simulink model "B12U_HVDC"  (R2024a)
settings: Solver=VariableStepAuto  StartTime=0.0  StopTime=0.02  MaxStep=1e-5  RelTol=1e-3
undefined symbols (not defined in the file or in its folder): D1, Delta
libraries: spsDiodeLib x12, spsVoltageMeasurementLib x7, spsACVoltageSourceLib x3, spsCurrentMeasurementLib x1, spsGroundLib x1, spsSeriesRLCBranchLib x1, spsThreePhaseTransformerThreeWindingsLib x1, sps_lib x1
settings Model: Creator=E370_  LastModifiedBy=E370_

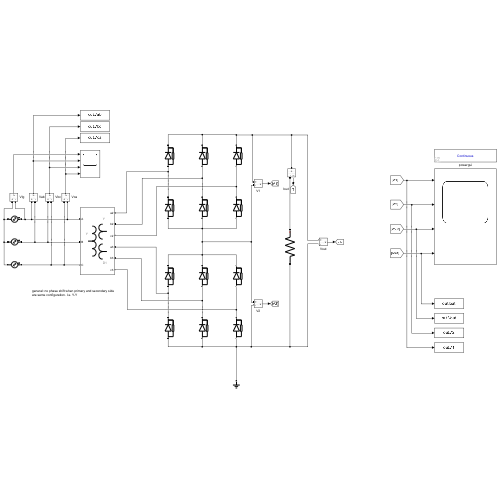
[thumbnail: Simulink's stored preview of the top-level diagram]
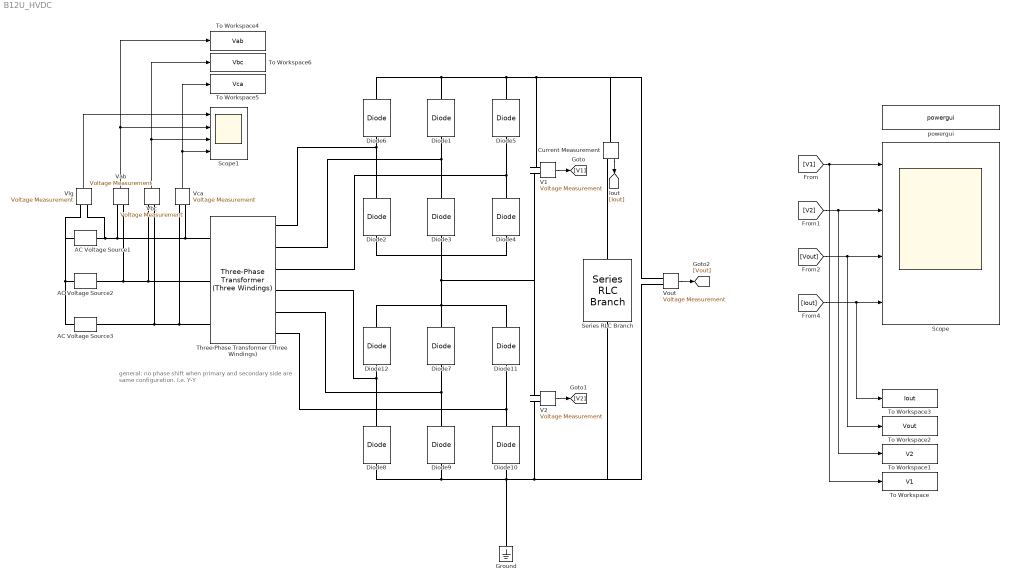
== system B12U_HVDC ==
  note: general: no phase shift when primary and secondary side
      | are same configuration. I.e. Y-Y
  AC Voltage Source1 : spsACVoltageSourceLib/AC Voltage Source  Amplitude=220  Phase=0  Frequency=50  SampleTime=0  Measurements=None  BusType=swing  Pref=10e3  Qref=0  Qmin=-inf  Qmax=+inf
  AC Voltage Source2 : spsACVoltageSourceLib/AC Voltage Source  Amplitude=220  Phase=-120  Frequency=50  SampleTime=0  Measurements=None  BusType=swing  Pref=10e3  Qref=0  Qmin=-inf  Qmax=+inf
  AC Voltage Source3 : spsACVoltageSourceLib/AC Voltage Source  Amplitude=220  Phase=-240  Frequency=50  SampleTime=0  Measurements=None  BusType=swing  Pref=10e3  Qref=0  Qmin=-inf  Qmax=+inf
  Current Measurement : spsCurrentMeasurementLib/Current Measurement  PhasorSimulation=off  OutputType=Complex  PSBequivalent=0
  Diode{1..12} (12 alike) : spsDiodeLib/Diode  Ron=0.001  Lon=0  Vf=0.0  IC=0  UseSnubber=0  Rs=500  Cs=250e-9  Measurements=off
  Ground : spsGroundLib/Ground  LConnTagsString=a
  Scope : Scope  NumInputPorts=4
  Scope1 : Scope  NumInputPorts=4
  Series RLC Branch : spsSeriesRLCBranchLib/Series RLC Branch  LConnTagsString=__new0  RConnTagsString=__new0  BranchType=R  Resistance=1  Inductance=0.02  SetiL0=off  InitialCurrent=0  Capacitance=1e-6  Setx0=off  InitialVoltage=0  Measurements=None
  Three-Phase Transformer (Three Windings) : spsThreePhaseTransformerThreeWindingsLib/Three-Phase Transformer (Three Windings)  Winding1Connection=Y  Winding2Connection=Y  Winding3Connection=Delta (D1)  CoreType=Three single-phase transformers  SetSaturation=off  Hysteresis=off  DataFile='hysteresis'  SetInitialFlux=off  Measurements=None  UNITS=pu  NominalPower=[ 250e6 , 50 ]  Winding1=[300 0.02 0]  Winding2=[100 0.02 0]  Winding3=[100 0.02 0]  Rm=500  Lm=500  L0=0.5  Saturation=[ 0,0 ; 0.0024,1.2 ; 1.0,1.52 ]  InitialFluxes=[0.8 -0.8 0.7]  BreakLoop=off  DiscreteSolver=Trapezoidal iterative  DataType=off  TransfoNumber=1
      settings: LibrarySourceBlock=|
      | sps_lib/Power Grid Elements/Three-Phase
      | Transformer
      | (Three Windings)
  To Workspace : ToWorkspace  VariableName=V1  SaveFormat=Timeseries  SampleTime=-1
  To Workspace1 : ToWorkspace  VariableName=V2  SaveFormat=Timeseries  SampleTime=-1
  To Workspace2 : ToWorkspace  VariableName=Vout  SaveFormat=Timeseries  SampleTime=-1
  To Workspace3 : ToWorkspace  VariableName=Iout  SaveFormat=Timeseries  SampleTime=-1
  To Workspace4 : ToWorkspace  VariableName=Vab  SaveFormat=Timeseries  SampleTime=-1
  To Workspace5 : ToWorkspace  VariableName=Vca  SaveFormat=Timeseries  SampleTime=-1
  To Workspace6 : ToWorkspace  VariableName=Vbc  SaveFormat=Timeseries  SampleTime=-1
  V1 : spsVoltageMeasurementLib/Voltage Measurement  PhasorSimulation=off  OutputType=Complex  PSBequivalent=0
  V2 : spsVoltageMeasurementLib/Voltage Measurement  PhasorSimulation=off  OutputType=Complex  PSBequivalent=0
  Vab : spsVoltageMeasurementLib/Voltage Measurement  PhasorSimulation=off  OutputType=Complex  PSBequivalent=0
  Vbc : spsVoltageMeasurementLib/Voltage Measurement  PhasorSimulation=off  OutputType=Complex  PSBequivalent=0
  Vca : spsVoltageMeasurementLib/Voltage Measurement  PhasorSimulation=off  OutputType=Complex  PSBequivalent=0
  Vlg : spsVoltageMeasurementLib/Voltage Measurement  PhasorSimulation=off  OutputType=Complex  PSBequivalent=0
  Vout : spsVoltageMeasurementLib/Voltage Measurement  PhasorSimulation=off  OutputType=Complex  PSBequivalent=0
  powergui : sps_lib/powergui  Priority=1  SimulationMode=Continuous  SampleTime=50e-6  frequency=60  Iterations=50  frequencyindice=50  Pbase=100e6  ErrMax=1e-4  UnitsV=kV  UnitsW=MW  buscounter=0  FunctionMessages=off  echomessages=off  EnableUseOfTLC=off  CurrentSourceSwitches=off  DisableSnubberDevices=off  DisableRonSwitches=off  DisableVfSwitches=off  DisplayEquations=off  AutomaticDiscreteSolvers=off  SolverType=Tustin/Backward Euler (TBE)  Interpol=off  ExternalGateDelay=off  methode=off  Ts=100  x0status=blocks  SPID=on  SwTol=0  HookPort=off  NonlinearTolerance=1e-4  nMaxIteration=100  ContinueOnMaxIteration=off  RestoreLinks=warning  ResistiveCurrentMeasurement=off  Frange=[0:2:500]  Ylog=off  Xlog=on  ShowGrid=off  save=off  variable=ZData  structure=0  ZoomFFT=off  StartTime=0.0  cycles=1  DisplayStyle=1  fundamental=60  FreqAxis=off  MaxFrequency=1000  frequencyindicesteady=1  RmsSteady=1  display=off
  wires:
  V1/1 -> [V1]
  V2/1 -> [V2]
  Vout/1 -> [Vout]
  [V1] -> To Workspace/1, Scope/1
  [V2] -> To Workspace1/1, Scope/2
  [Vout] -> To Workspace2/1, Scope/3
  Vlg/1 -> Scope1/1
  Vab/1 -> Scope1/2, To Workspace4/1
  [Iout] -> To Workspace3/1, Scope/4
  Vbc/1 -> To Workspace6/1, Scope1/3
  Vca/1 -> To Workspace5/1, Scope1/4
  Current Measurement/1 -> [Iout]
  connections:
  Diode6/LConn1 -- Three-Phase Transformer (Three Windings)/RConn1 -- Diode2/RConn1
  Diode1/LConn1 -- Three-Phase Transformer (Three Windings)/RConn2 -- Diode3/RConn1
  Diode5/LConn1 -- Three-Phase Transformer (Three Windings)/RConn3 -- Diode4/RConn1
  Diode5/RConn1 -- Vout/LConn1 -- Current Measurement/LConn1 -- V1/LConn1 -- Diode1/RConn1 -- Diode6/RConn1
  Diode11/RConn1 -- V2/LConn1 -- V1/LConn2 -- Diode3/LConn1 -- Diode4/LConn1 -- Diode2/LConn1 -- Diode7/RConn1 -- Diode12/RConn1
  Diode8/LConn1 -- Diode9/LConn1 -- Ground/LConn1 -- V2/LConn2 -- Series RLC Branch/RConn1 -- Vout/LConn2 -- Diode10/LConn1
  Diode12/LConn1 -- Three-Phase Transformer (Three Windings)/RConn4 -- Diode8/RConn1
  Diode7/LConn1 -- Diode9/RConn1 -- Three-Phase Transformer (Three Windings)/RConn5
  Diode11/LConn1 -- Three-Phase Transformer (Three Windings)/RConn6 -- Diode10/RConn1
  AC Voltage Source1/RConn1 -- Vca/LConn2 -- Three-Phase Transformer (Three Windings)/LConn1 -- Vab/LConn1 -- Vlg/LConn2
  AC Voltage Source2/RConn1 -- Vbc/LConn1 -- Three-Phase Transformer (Three Windings)/LConn2 -- Vab/LConn2
  AC Voltage Source3/RConn1 -- Vbc/LConn2 -- Vca/LConn1 -- Three-Phase Transformer (Three Windings)/LConn3
  AC Voltage Source2/LConn1 -- Vlg/LConn1 -- AC Voltage Source1/LConn1 -- AC Voltage Source3/LConn1
  Series RLC Branch/LConn1 -- Current Measurement/RConn1
